simulink model "pendulum_sim"  (R2016b)
settings: Solver=ode45  StartTime=0.0  StopTime=300  RelTol=1e-3  EnableMultiTasking=on
InitFcn:
  | addpath ./..
  | pendulum_param
  | pendulumParamHW12
undefined symbols (not defined in the file or in its folder): P, pendulum_animation, pendulum_ctrl
settings Model: Creator=beard  LastModifiedBy=mclain
settings DataIOCC: LimitDataPoints=on  SaveFormat=Array  SignalLoggingSaveFormat=ModelDataLogs
settings OptimizationCC: ExpressionDepthLimit=2147483647  InitFltsAndDblsToZero=on  LifeSpan=inf
settings DebuggingCC: UnderspecifiedInitializationDetection=Classic  MergeDetectMultiDrivingBlocksExec=none  SolverPrmCheckMsg=warning  FcnCallInpInsideContextMsg=warning  StateNameClashWarn=warning  SFUnexpectedBacktrackingDiag=warning  SFNoUnconditionalDefaultTransitionDiag=warning  SFExecutionAtInitializationDiag=none
settings HardwareCC: ProdBitPerPointer=32  ProdBitPerSizeT=32  ProdBitPerPtrDiffT=32  ProdLargestAtomicFloat=None  ProdIntDivRoundTo=Undefined  ProdEndianess=Unspecified  ProdWordSize=32  ProdHWDeviceType=32-bit Generic
settings ModelReferenceCC: PropagateSignalLabelsOutOfModel=off
settings GRTTargetCC: TargetLangStandard=C89/C90 (ANSI)  GeneratePreprocessorConditionals=Disable all  CombineOutputUpdateFcns=off  GRTInterface=on
settings ConfigComp: CovMetricSettings=dw  CovHtmlReporting=on  CovSaveCumulativeToWorkspaceVar=on  CovSaveSingleToWorkspaceVar=on  CovExternalEMLEnable=off

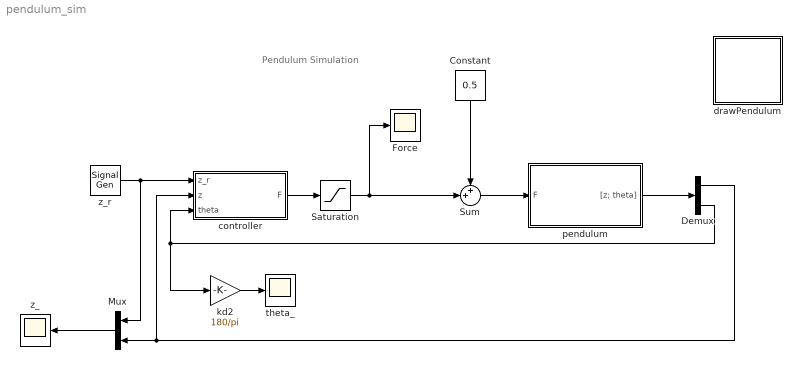
== system pendulum_sim ==
  note: Pendulum Simulation
  Constant : Constant  Value=0.5
  Demux : Demux  Outputs=2
  Force : Scope
  Mux : Mux  Inputs=2
  Saturation : Saturate  UpperLimit=P.F_max  LowerLimit=-P.F_max
  Sum : Sum  Inputs=++|
  controller : Subsystem
  drawPendulum : Subsystem
      mask Display: image(imread('tv.jpg'))
  kd2 : Gain  Gain=180/pi
  pendulum : Subsystem
  theta_ : Scope
  z_ : Scope
  z_r : SignalGenerator  WaveForm=square  Amplitude=0.5  Frequency=0.05
  wires:
  pendulum/1("[z; theta]") -> Demux/1
  controller/1(F) -> Saturation/1
  Saturation/1 -> Sum/2, Force/1
  Demux/2 -> controller/3(theta), kd2/1
  Demux/1 -> Mux/2, controller/2(z)
  z_r/1 -> Mux/1, controller/1(z_r)
  Mux/1 -> z_/1
  kd2/1 -> theta_/1
  Sum/1 -> pendulum/1(F)
  Constant/1 -> Sum/1

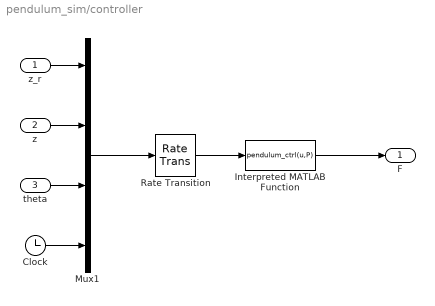
== system pendulum_sim/controller ==
  z_r : Inport
  z : Inport  Port=2
  theta : Inport  Port=3
  Clock : Clock
  Interpreted MATLAB Function : MATLABFcn  MATLABFcn=pendulum_ctrl(u,P)  OutputDimensions=1
  Mux1 : Mux
  Rate Transition : RateTransition  OutPortSampleTime=P.Ts
  F : Outport
  wires:
  Mux1/1 -> Rate Transition/1
  z_r/1 -> Mux1/1
  Interpreted MATLAB Function/1 -> F/1
  Clock/1 -> Mux1/4
  Rate Transition/1 -> Interpreted MATLAB Function/1
  theta/1 -> Mux1/3
  z/1 -> Mux1/2

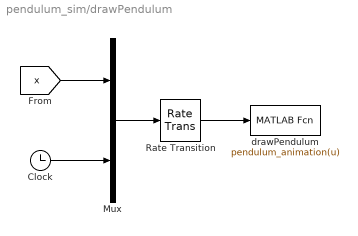
== system pendulum_sim/drawPendulum ==
  Clock : Clock
  Mux : Mux  Inputs=2
  Rate Transition : RateTransition  OutPortSampleTime=P.t_plot
  drawPendulum : MATLABFcn  MATLABFcn=pendulum_animation(u)  OutputDimensions=0
  wires:
  Mux/1 -> Rate Transition/1
  [x] -> Mux/1
  Clock/1 -> Mux/2
  Rate Transition/1 -> drawPendulum/1

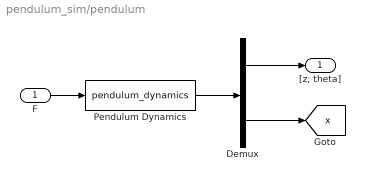
== system pendulum_sim/pendulum ==
  F : Inport
  Demux : Demux  Outputs=[2;4]
  Pendulum Dynamics : S-Function  FunctionName=pendulum_dynamics  Parameters=P  SFunctionDeploymentMode=off  EnableBusSupport=off
  "[z; theta]" : Outport
  tag scope: x=global
  wires:
  F/1 -> Pendulum Dynamics/1
  Pendulum Dynamics/1 -> Demux/1
  Demux/1 -> "[z; theta]"/1
  Demux/2 -> [x]
